simulink model "joystick"  (R2021b)
settings: Solver=FixedStepAuto  StartTime=0.0  StopTime=3  RelTol=1e-3
libraries: arduinomotorcarrierlib x2, arduinolib x2, arduinoethernetlib x1, arduinowifilib x1
settings Model: ExtModeTrigDuration=2  Creator=cirie  LastModifiedBy=cirie
settings OptimizationCC: EnhancedBackFolding=on  PassReuseOutputArgsAs=Individual arguments  ZeroExternalMemoryAtStartup=off  ZeroInternalMemoryAtStartup=off  MaxStackSize=64  OptimizeBlockOrder=speed  DifferentSizesBufferReuse=on  OptimizationCustomize=off  EfficientTunableParamExpr=on
settings DebuggingCC: ParameterTunabilityLossMsg=error
settings HardwareCC: ProdBitPerPointer=32  ProdBitPerSizeT=32  ProdBitPerPtrDiffT=32  ProdLargestAtomicInteger=Long  ProdLargestAtomicFloat=Double  ProdWordSize=32  ProdHWDeviceType=ARM Compatible->ARM Cortex
settings SFSimCC: MATLABDynamicMemAlloc=off
settings RTWCC: Description=Embedded Coder  SystemTargetFile=ert.tlc  HardwareBoard=Arduino MKR WiFi 1010  TemplateMakefile=ert_default_tmf  Toolchain=Arduino ARM
settings CodeAppCC: ForceParamTrailComments=on  IgnoreCustomStorageClasses=off  OperatorAnnotations=on  SimulinkDataObjDesc=on  SFDataObjDesc=on  InsertBlockDesc=on
settings ERTTargetCC: SupportContinuousTime=on  SupportVariableSizeSignals=on  ExtModeTransport=3  ExtModeStaticAlloc=on  ExtModeStaticAllocSize=8192  ExtModeMexFile=ext_xcp  ExtModeIntrfLevel=Level2 - Open

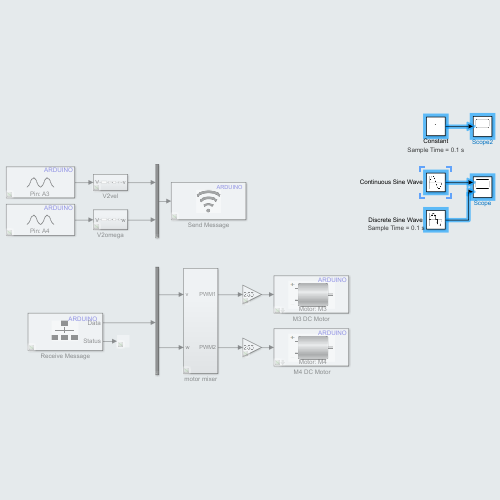
[thumbnail: Simulink's stored preview of the top-level diagram]
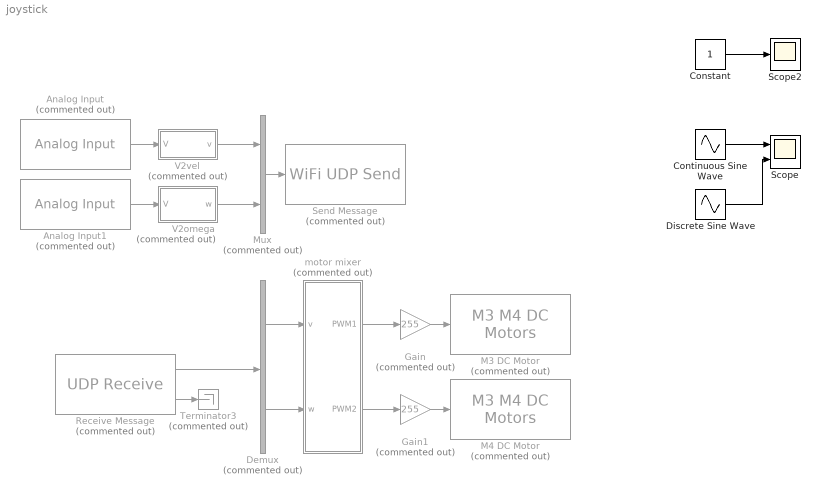
== system joystick ==
  " M4 DC Motor" : arduinomotorcarrierlib/M3 M4 DC Motors  Commented=on  MotorNumber=M4  forwardPinNumber=4  reversePinNumber=5
      settings: SourceProductBaseCode=ARDUINO
  Analog Input : arduinolib/Analog Input  Commented=on  pinNumber=3  ReadResultsOnly=off  ConversionTriggerSource=Software  ExternalTriggerType=uint32( 0 )  OutputDataType=uint16  EnableConversionCompleteNotify=off  EnableOuputStatus=off  SampleTime=-1  blockPlatform=arduino
  Analog Input1 : arduinolib/Analog Input  Commented=on  pinNumber=4  ReadResultsOnly=off  ConversionTriggerSource=Software  ExternalTriggerType=uint32( 0 )  OutputDataType=uint16  EnableConversionCompleteNotify=off  EnableOuputStatus=off  SampleTime=-1  blockPlatform=arduino
  Constant : Constant  SampleTime=0.1
      settings: AttributesFormatString=Sample Time = %<SampleTime> s
  Continuous Sine Wave : Sin  Frequency=5  SampleTime=0
  Demux : Demux  Commented=on  Outputs=2
  Discrete Sine Wave : Sin  Frequency=5  SampleTime=0.1
      settings: AttributesFormatString=Sample Time = %<SampleTime> s
  Gain : Gain  Commented=on  Gain=255
  Gain1 : Gain  Commented=on  Gain=255
  M3 DC Motor : arduinomotorcarrierlib/M3 M4 DC Motors  Commented=on  MotorNumber=M3  forwardPinNumber=3  reversePinNumber=2
      settings: SourceProductBaseCode=ARDUINO
  Mux : Mux  Commented=on  Inputs=2
  Receive Message : arduinoethernetlib/UDP Receive  Commented=on  localport=56789  sampleTime=1  blockPlatform=arduino  UDP_IDX=0  port_array_ordered=0
      settings: SourceProductBaseCode=ARDUINO
  Scope : Scope  NumInputPorts=2
  Scope2 : Scope
  Send Message : arduinowifilib/WiFi UDP Send  Commented=on  remoteIPOctetString=192.168.1.2  remoteport=50002  localport=50001  remoteipoctet1=192  remoteipoctet2=168  remoteipoctet3=1  remoteipoctet4=2  wifiUDPIndex=0  blockPlatform=ARDUINO  isARMArch=false
      settings: SourceProductBaseCode=ARDUINO
  Terminator3 : Terminator  Commented=on
  V2omega : Subsystem  Commented=on
  V2vel : Subsystem  Commented=on
  motor mixer : Subsystem  Commented=on
  wires:
  V2vel/1(v) -> Mux/1
  V2omega/1(w) -> Mux/2
  Mux/1 -> Send Message/1
  Analog Input/1 -> V2vel/1(V)
  Analog Input1/1 -> V2omega/1(V)
  Receive Message/2 -> Terminator3/1
  Receive Message/1 -> Demux/1
  Demux/1 -> motor mixer/1(v)
  Demux/2 -> motor mixer/2(w)
  motor mixer/1(PWM1) -> Gain/1
  Gain/1 -> M3 DC Motor/1
  Gain1/1 -> " M4 DC Motor"/1
  motor mixer/2(PWM2) -> Gain1/1
  Constant/1 -> Scope2/1
  Continuous Sine Wave/1 -> Scope/1
  Discrete Sine Wave/1 -> Scope/2

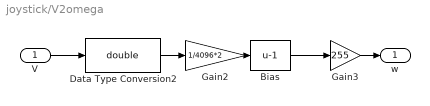
== system joystick/V2omega ==
  V : Inport
  Bias : Bias  Bias=-1
  Data Type Conversion2 : DataTypeConversion  OutDataTypeStr=double
  Gain2 : Gain  Gain=1/4096*2
  Gain3 : Gain  Gain=255
  w : Outport
  wires:
  Gain3/1 -> w/1
  Gain2/1 -> Bias/1
  V/1 -> Data Type Conversion2/1
  Data Type Conversion2/1 -> Gain2/1
  Bias/1 -> Gain3/1

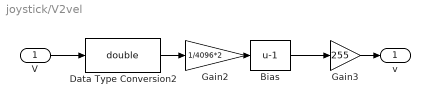
== system joystick/V2vel ==
  V : Inport
  Bias : Bias  Bias=-1
  Data Type Conversion2 : DataTypeConversion  OutDataTypeStr=double
  Gain2 : Gain  Gain=1/4096*2
  Gain3 : Gain  Gain=255
  v : Outport
  wires:
  Bias/1 -> Gain3/1
  Data Type Conversion2/1 -> Gain2/1
  V/1 -> Data Type Conversion2/1
  Gain2/1 -> Bias/1
  Gain3/1 -> v/1

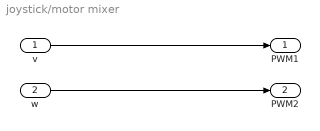
== system joystick/motor mixer ==
  v : Inport
  w : Inport  Port=2
  PWM1 : Outport
  PWM2 : Outport  Port=2
  wires:
  v/1 -> PWM1/1
  w/1 -> PWM2/1
